simulink model "MidSideProcessor_Start"  (R2025b)
settings: Solver=FixedStepDiscrete  StopTime=10
libraries: dspsnks4 x1, dspvision x1
settings Model: Creator=Adam  LastModifiedBy=skerber
settings SolverCC: AlgebraicLoopSolver=TrustRegion  AutoInsertRateTranBlk=on
settings DataIOCC: LimitDataPoints=on  SaveOutput=off  SignalLogging=off  SaveTime=off
settings OptimizationCC: LifeSpan=inf
settings DebuggingCC: AlgebraicLoopMsg=error  SingleTaskRateTransMsg=error  UnconnectedInputMsg=warning  UnconnectedOutputMsg=warning  UnconnectedLineMsg=warning  AllowSymbolicDim=off  SFUnexpectedBacktrackingDiag=warning  SFNoUnconditionalDefaultTransitionDiag=warning  SFExecutionAtInitializationDiag=none  ArithmeticOperatorsInVariantConditions=warning
settings ModelReferenceCC: EnableRefExpFcnMdlSchedulingChecks=on
settings SFSimCC: SimUseLocalCustomCode=off  CustomCodeUndefinedFunction=UseInterfaceOnly
settings RTWCC: RTWUseLocalCustomCode=off  GPUComputeCapability=3.5  DLArmComputeVersion=19.05
settings CodeAppCC: StateflowObjectComments=on
settings GRTTargetCC: TargetLangStandard=C89/C90 (ANSI)
settings ConfigComp: CovMetricSettings=dw  CovSaveCumulativeToWorkspaceVar=on  CovSaveSingleToWorkspaceVar=on  CovExternalEMLEnable=off  CovSFcnEnable=off

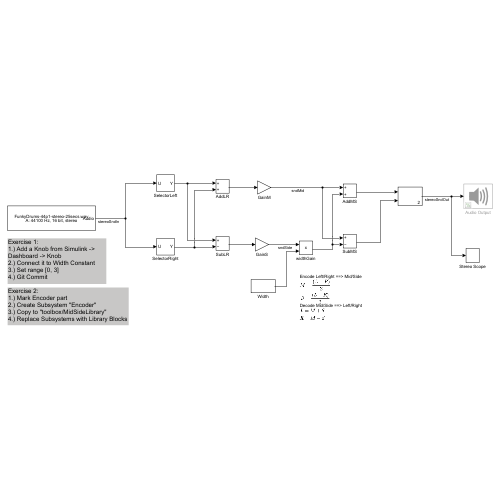
[thumbnail: Simulink's stored preview of the top-level diagram]
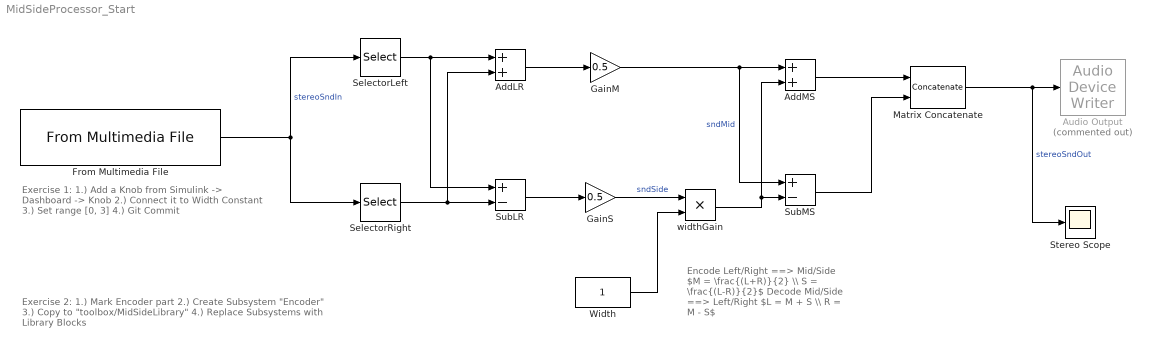
== system MidSideProcessor_Start ==
  note: Exercise 1:
      | 1.) Add a Knob from Simulink -> Dashboard -> Knob
      | 2.) Connect it to Width Constant
      | 3.) Set range [0, 3]
      | 4.) Git Commit
  note: Encode Left/Right ==> Mid/Side
      | $M = \frac{(L+R)}{2} \\ S = \frac{(L-R)}{2}$
      | Decode Mid/Side ==> Left/Right
      | $L = M + S \\ R = M - S$
  note: Exercise 2:
      | 1.) Mark Encoder part
      | 2.) Create Subsystem "Encoder"
      | 3.) Copy to "toolbox/MidSideLibrary"
      | 4.) Replace Subsystems with Library Blocks
  AddLR : Sum
  AddMS : Sum
  Audio Output : dspsnks4/Audio Device Writer  Commented=on  Driver=DirectSound  Device=Default  InheritSampleRate=on  SampleRate=44100  BitDepth=16-bit integer  BufferSize=4096  NumBuffers=10  DefaultOutputChannelMapping=on  OutputChannelMapping=1:2  OutputNumUnderrunSamples=off  DriverIdx=1  DeviceWarnFlag=''
  From Multimedia File : dspvision/From Multimedia File  inputFilename=FunkyDrums-44p1-stereo-25secs.wav  readRange=[1 Inf]  loop=on  numPlays=inf  outputStreams=Audio only  videoDataType=single  audioDataType=double  inheritSampleTime=on  userDefinedSampleTime=1/30  noAudioOutput=off  isIntensityVideo=off  fourcc=RGB  colorVideoFormat=Separate color signals  outputEOF=off  dataOrg=Column-major  audioFrameSize=1024  computeAudioFrameSize=off  outSamplingMode=Sample based
  GainM : Gain  Gain=0.5
  GainS : Gain  Gain=0.5
  Matrix Concatenate : Concatenate  Mode=Multidimensional array  ConcatenateDimension=2
  SelectorLeft : Selector  NumberOfDimensions=2  InputPortWidth=3  IndexOptions=Select all,Index vector (dialog)  Indices=[1 3],1  OutputSizes=1,1
  SelectorRight : Selector  NumberOfDimensions=2  InputPortWidth=3  IndexOptions=Select all,Index vector (dialog)  Indices=[1 3],2  OutputSizes=1,1
  Stereo Scope : Scope
      settings: TimeUnits=Metric (based on Time Span)  ActiveDisplayYMinimum=-0.854809564433882  ActiveDisplayYMaximum=1.0535340538460525  YLabel=Amplitude
  SubLR : Sum  Inputs=+-
  SubMS : Sum  Inputs=+-
  Width : Constant
  widthGain : Product
  wires:
  Width/1 -> widthGain/2
  AddLR/1 -> GainM/1
  AddMS/1 -> Matrix Concatenate/1
  GainM/1 -> AddMS/1, SubMS/1  "sndMid"
  SelectorLeft/1 -> AddLR/1, SubLR/1
  SelectorRight/1 -> AddLR/2, SubLR/2
  SubLR/1 -> GainS/1
  SubMS/1 -> Matrix Concatenate/2
  From Multimedia File/1 -> SelectorLeft/1, SelectorRight/1  "stereoSndIn"
  GainS/1 -> widthGain/1  "sndSide"
  Matrix Concatenate/1 -> Audio Output/1, Stereo Scope/1  "stereoSndOut"
  widthGain/1 -> AddMS/2, SubMS/2
